simulink model "ControleFF_D_NL"  (R2020b)
settings: Solver=FixedStepAuto  StartTime=0  StopTime=10  FixedStep=1e-3  RelTol=1e-3
values from neighbouring files (symbols this model uses):
  alpha = alpha_vec(l)    [kermani_parameters.m]    (also in teste_controle_nao_linear.m = 1.25)
  Beff = 1    [kermani_parameters.m]    (also in teste_controle_nao_linear.m = 50)
  Fc = Fc_vec(k)    [kermani_parameters.m]    (also in teste_controle_nao_linear.m = 2173.5)
  Fs = Fs_vec(j)    [kermani_parameters.m]    (also in teste_controle_nao_linear.m = 2673.5)
  Jeff = 0.5    [kermani_parameters.m]    (also in teste_controle_nao_linear.m)
  K = (90/12)*(2*pi/60)    (= 0.785398163397)    [kermani_parameters.m]    (also in teste_controle_nao_linear.m)
  Kd = (2*xi*wn*Jeff - Beff)/K    (= 17.8253536263)    [kermani_parameters.m]    (also in teste_controle_nao_linear.m = -44.5633840657)
  Kp = (wn^2*Jeff)/K    (= 143.239448783)    [kermani_parameters.m]    (also in teste_controle_nao_linear.m)
  N = 3    [kermani_parameters.m]    (also in teste_controle_nao_linear.m)
  phi = 43.47    [teste_controle_nao_linear.m]
  r = 1./[231.22*4 139.138 139.138 231.22 231.22]    [kermani_parameters.m]    (also in teste_controle_nao_linear.m)
  sigma0 = sigma0_vec(m)    [kermani_parameters.m]    (also in teste_controle_nao_linear.m = 10000)
  sigma1 = sigma1_vec(n)    [kermani_parameters.m]    (also in teste_controle_nao_linear.m = 1000)
  sigma2 = sigma2_vec(o)    [kermani_parameters.m]    (also in teste_controle_nao_linear.m = 10)
libraries: simulink_extras x21
(part 11 of 14)

== matlab function ControleFF_D_NL/Dinâmica do robô2/Perturbação/V1 ==
  data: Th input; V output; dTh input
function V = calcul_V(Th, dTh)

th1 = Th(1);
th2 = Th(2);
th3 = Th(3);
th4 = Th(4);
th5 = Th(5);
dth1 = dTh(1);
dth2 = dTh(2);
dth3 = dTh(3);
dth4 = dTh(4);
dth5 = dTh(5);

V = [((217*cos(th2)*cos(th3)*cos(th4)*sin(th4))/80000 - (217*cos(th4)*sin(th2)*sin(th3)*sin(th4))/80000 + (87*cos(th2)*sin(th3)*sin(th4)*sin(th5))/5000 + (87*cos(th3)*sin(th2)*sin(th4)*sin(th5))/5000 + (9*cos(th2)*cos(th5)*sin(th3)*sin(th4)*sin(th5))/3200 + (9*cos(th3)*cos(th5)*sin(th2)*sin(th4)*sin(th5))/3200 - (9*cos(th2)*cos(th3)*cos(th4)*cos(th5)^2*sin(th4))/3200 + (9*cos(th4)*cos(th5)^2*sin(th2)*sin(th3)*sin(th4))/3200)*dth3^2 + ((217*cos(th2)*cos(th3)*cos(th4)*sin(th4))/80000 - (3*cos(th2)*sin(th4)*sin(th5))/160 - (217*cos(th4)*sin(th2)*sin(th3)*sin(th4))/80000 + (87*cos(th2)*sin(th3)*sin(th4)*sin(th5))/5000 + (87*cos(th3)*sin(th2)*sin(th4)*sin(th5))/5000 + (9*cos(th2)*cos(th5)*sin(th3)*sin(th4)*sin(th5))/3200 + (9*cos(th3)*cos(th5)*sin(th2)*sin(th4)*sin(th5))/3200 - (9*cos(th2)*cos(th3)*cos(th4)*cos(th5)^2*sin(th4))/3200 + (9*cos(th4)*cos(th5)^2*sin(th2)*sin(th3)*sin(th4))/3200)*dth2^2 + ((217*cos(th2)*cos(th4)^2*sin(th3))/40000 - (353*cos(th3)*sin(th2))/40000 - (353*cos(th2)*sin(th3))/40000 + (217*cos(th3)*cos(th4)^2*sin(th2))/40000 + (9*cos(th2)*cos(th5)^2*sin(th3))/1600 + (9*cos(th3)*cos(th5)^2*sin(th2))/1600 - (9*cos(th2)*cos(th4)^2*cos(th5)^2*sin(th3))/1600 - (9*cos(th3)*cos(th4)^2*cos(th5)^2*sin(th2))/1600)*dth2*dth4 + ((217*cos(th2)*cos(th4)^2*sin(th3))/40000 - (353*cos(th3)*sin(th2))/40000 - (353*cos(th2)*sin(th3))/40000 + (217*cos(th3)*cos(th4)^2*sin(th2))/40000 + (9*cos(th2)*cos(th5)^2*sin(th3))/1600 + (9*cos(th3)*cos(th5)^2*sin(th2))/1600 - (9*cos(th2)*cos(th4)^2*cos(th5)^2*sin(th3))/1600 - (9*cos(th3)*cos(th4)^2*cos(th5)^2*sin(th2))/1600)*dth3*dth4 + ((217*cos(th2)*cos(th3)*cos(th4)*sin(th4))/40000 - (217*cos(th4)*sin(th2)*sin(th3)*sin(th4))/40000 + (87*cos(th2)*sin(th3)*sin(th4)*sin(th5))/2500 + (87*cos(th3)*sin(th2)*sin(th4)*sin(th5))/2500 + (9*cos(th2)*cos(th5)*sin(th3)*sin(th4)*sin(th5))/1600 + (9*cos(th3)*cos(th5)*sin(th2)*sin(th4)*sin(th5))/1600 - (9*cos(th2)*cos(th3)*cos(th4)*cos(th5)^2*sin(th4))/1600 + (9*cos(th4)*cos(th5)^2*sin(th2)*sin(th3)*sin(th4))/1600)*dth2*dth3 + ((217*cos(th2)^2*cos(th4)*sin(th4))/40000 + (217*cos(th3)^2*cos(th4)*sin(th4))/40000 + (3*cos(th2)^2*cos(th3)*sin(th4)*sin(th5))/80 - (217*cos(th2)^2*cos(th3)^2*cos(th4)*sin(th4))/20000 - (9*cos(th2)^2*cos(th4)*cos(th5)^2*sin(th4))/1600 - (9*cos(th3)^2*cos(th4)*cos(th5)^2*sin(th4))/1600 + (87*cos(th2)*sin(th2)*sin(th4)*sin(th5))/2500 + (87*cos(th3)*sin(th3)*sin(th4)*sin(th5))/2500 + (9*cos(th2)^2*cos(th3)^2*cos(th4)*cos(th5)^2*sin(th4))/800 + (9*cos(th2)*cos(th5)*sin(th2)*sin(th4)*sin(th5))/1600 + (9*cos(th3)*cos(th5)*sin(th3)*sin(th4)*sin(th5))/1600 - (3*cos(th2)*sin(th2)*sin(th3)*sin(th4)*sin(th5))/80 - (87*cos(th2)*cos(th3)^2*sin(th2)*sin(th4)*sin(th5))/1250 - (87*cos(th2)^2*cos(th3)*sin(th3)*sin(th4)*sin(th5))/1250 + (217*cos(th2)*cos(th3)*cos(th4)*sin(th2)*sin(th3)*sin(th4))/20000 - (9*cos(th2)*cos(th3)^2*cos(th5)*sin(th2)*sin(th4)*sin(th5))/800 - (9*cos(th2)^2*cos(th3)*cos(th5)*sin(th3)*sin(th4)*sin(th5))/800 - (9*cos(th2)*cos(th3)*cos(th4)*cos(th5)^2*sin(th2)*sin(th3)*sin(th4))/800)*dth1*dth4 + ((87*cos(th4)*sin(th5))/2500 - (8453*sin(2*th3))/31250 - (8453*sin(2*th2))/31250 - (33*cos(th2)^2*cos(th3))/50 - (87*cos(th2)*cos(th5)*sin(th2))/1250 - (87*cos(th3)*cos(th5)*sin(th3))/1250 + (9*cos(th4)*cos(th5)*sin(th5))/1600 + (33*cos(th2)*sin(th2)*sin(th3))/50 - (3*cos(th2)^2*cos(th3)*cos(th5))/80 + (16906*cos(th2)*cos(th3)^2*sin(th2))/15625 + (217*cos(th2)*cos(th4)^2*sin(th2))/40000 + (16906*cos(th2)^2*cos(th3)*sin(th3))/15625 - (9*cos(th2)*cos(th5)^2*sin(th2))/1600 + (217*cos(th3)*cos(th4)^2*sin(th3))/40000 - (9*cos(th3)*cos(th5)^2*sin(th3))/1600 - (87*cos(th2)^2*cos(th4)*sin(th5))/1250 - (87*cos(th3)^2*cos(th4)*sin(th5))/1250 + (3*cos(th2)^2*cos(th4)*sin(th3)*sin(th5))/80 - (217*cos(th2)*cos(th3)^2*cos(th4)^2*sin(th2))/20000 + (9*cos(th2)*cos(th3)^2*cos(th5)^2*sin(th2))/800 - (217*cos(th2)^2*cos(th3)*cos(th4)^2*sin(th3))/20000 - (9*cos(th2)*cos(th4)^2*cos(th5)^2*sin(th2))/1600 + (9*cos(th2)^2*cos(th3)*cos(th5)^2*sin(th3))/800 + (87*cos(th2)^2*cos(th3)^2*cos(th4)*sin(th5))/625 - (9*cos(th3)*cos(th4)^2*cos(th5)^2*sin(th3))/1600 + (3*cos(th2)*cos(th5)*sin(th2)*sin(th3))/80 + (87*cos(th2)*cos(th3)^2*cos(th5)*sin(th2))/625 + (87*cos(th2)^2*cos(th3)*cos(th5)*sin(th3))/625 - (9*cos(th2)^2*cos(th4)*cos(th5)*sin(th5))/800 - (9*cos(th3)^2*cos(th4)*cos(th5)*sin(th5))/800 + (9*cos(th2)*cos(th3)^2*cos(th4)^2*cos(th5)^2*sin(th2))/800 + (9*cos(th2)^2*cos(th3)*cos(th4)^2*cos(th5)^2*sin(th3))/800 + (9*cos(th2)^2*cos(th3)^2*cos(th4)*cos(th5)*sin(th5))/400 + (3*cos(th2)*cos(th3)*cos(th4)*sin(th2)*sin(th5))/80 - (87*cos(th2)*cos(th3)*cos(th4)*sin(th2)*sin(th3)*sin(th5))/625 - (9*cos(th2)*cos(th3)*cos(th4)*cos(th5)*sin(th2)*sin(th3)*sin(th5))/400)*dth1*dth3 + ((33*cos(th3))/50 - (53231*sin(2*th2))/62500 - (8453*sin(2*th3))/31250 + (87*cos(th4)*sin(th5))/2500 - (33*cos(th2)^2*cos(th3))/25 + (3*cos(th3)*cos(th5))/80 - (87*cos(th2)*cos(th5)*sin(th2))/1250 - (87*cos(th3)*cos(th5)*sin(th3))/1250 + (9*cos(th4)*cos(th5)*sin(th5))/1600 + (33*cos(th2)*sin(th2)*sin(th3))/25 - (3*cos(th4)*sin(th3)*sin(th5))/80 - (3*cos(th2)^2*cos(th3)*cos(th5))/40 + (16906*cos(th2)*cos(th3)^2*sin(th2))/15625 + (217*cos(th2)*cos(th4)^2*sin(th2))/40000 + (16906*cos(th2)^2*cos(th3)*sin(th3))/15625 - (9*cos(th2)*cos(th5)^2*sin(th2))/1600 + (217*cos(th3)*cos(th4)^2*sin(th3))/40000 - (9*cos(th3)*cos(th5)^2*sin(th3))/1600 - (87*cos(th2)^2*cos(th4)*sin(th5))/1250 - (87*cos(th3)^2*cos(th4)*sin(th5))/1250 + (3*cos(th2)^2*cos(th4)*sin(th3)*sin(th5))/40 - (217*cos(th2)*cos(th3)^2*cos(th4)^2*sin(th2))/20000 + (9*cos(th2)*cos(th3)^2*cos(th5)^2*sin(th2))/800 - (217*cos(th2)^2*cos(th3)*cos(th4)^2*sin(th3))/20000 - (9*cos(th2)*cos(th4)^2*cos(th5)^2*sin(th2))/1600 + (9*cos(th2)^2*cos(th3)*cos(th5)^2*sin(th3))/800 + (87*cos(th2)^2*cos(th3)^2*cos(th4)*sin(th5))/625 - (9*cos(th3)*cos(th4)^2*cos(th5)^2*sin(th3))/1600 + (3*cos(th2)*cos(th5)*sin(th2)*sin(th3))/40 + (87*cos(th2)*cos(th3)^2*cos(th5)*sin(th2))/625 + (87*cos(th2)^2*cos(th3)*cos(th5)*sin(th3))/625 - (9*cos(th2)^2*cos(th4)*cos(th5)*sin(th5))/800 - (9*cos(th3)^2*cos(th4)*cos(th5)*sin(th5))/800 + (9*cos(th2)*cos(th3)^2*cos(th4)^2*cos(th5)^2*sin(th2))/800 + (9*cos(th2)^2*cos(th3)*cos(th4)^2*cos(th5)^2*sin(th3))/800 + (9*cos(th2)^2*cos(th3)^2*cos(th4)*cos(th5)*sin(th5))/400 + (3*cos(th2)*cos(th3)*cos(th4)*sin(th2)*sin(th5))/40 - (87*cos(th2)*cos(th3)*cos(th4)*sin(th2)*sin(th3)*sin(th5))/625 - (9*cos(th2)*cos(th3)*cos(th4)*cos(th5)*sin(th2)*sin(th3)*sin(th5))/400)*dth1*dth2 + ((3*cos(th2)*sin(th4)*sin(th5))/160 - (87*cos(th2)*sin(th3)*sin(th4)*sin(th5))/5000 - (87*cos(th3)*sin(th2)*sin(th4)*sin(th5))/5000)*dth5^2 + ((3*cos(th2)*sin(th4)*sin(th5))/160 - (87*cos(th2)*sin(th3)*sin(th4)*sin(th5))/5000 - (87*cos(th3)*sin(th2)*sin(th4)*sin(th5))/5000 - (9*cos(th2)*cos(th5)*sin(th3)*sin(th4)*sin(th5))/3200 - (9*cos(th3)*cos(th5)*sin(th2)*sin(th4)*sin(th5))/3200)*dth4^2 + ((cos(th2)*cos(th4)*sin(th3))/625 - (3*cos(th2)*cos(th4)*cos(th5))/80 + (cos(th3)*cos(th4)*sin(th2))/625 + (87*cos(th2)*cos(th4)*cos(th5)*sin(th3))/2500 + (87*cos(th3)*cos(th4)*cos(th5)*sin(th2))/2500 + (9*cos(th2)*cos(th3)*cos(th5)*sin(th5))/1600 - (9*cos(th5)*sin(th2)*sin(th3)*sin(th5))/1600 + (9*cos(th2)*cos(th4)*cos(th5)^2*sin(th3))/1600 + (9*cos(th3)*cos(th4)*cos(th5)^2*sin(th2))/1600)*dth4*dth5 + ((289*cos(th2)*cos(th3)*sin(th4))/40000 - (289*sin(th2)*sin(th3)*sin(th4))/40000 + (9*cos(th5)^2*sin(th2)*sin(th3)*sin(th4))/1600 - (9*cos(th2)*cos(th3)*cos(th5)^2*sin(th4))/1600 + (9*cos(th2)*cos(th4)*cos(th5)*sin(th3)*sin(th4)*sin(th5))/1600 + (9*cos(th3)*cos(th4)*cos(th5)*sin(th2)*sin(th4)*sin(th5))/1600)*dth2*dth5 + ((289*cos(th2)*cos(th3)*sin(th4))/40000 - (289*sin(th2)*sin(th3)*sin(th4))/40000 + (9*cos(th5)^2*sin(th2)*sin(th3)*sin(th4))/1600 - (9*cos(th2)*cos(th3)*cos(th5)^2*sin(th4))/1600 + (9*cos(th2)*cos(th4)*cos(th5)*sin(th3)*sin(th4)*sin(th5))/1600 + (9*cos(th3)*cos(th4)*cos(th5)*sin(th2)*sin(th4)*sin(th5))/1600)*dth3*dth5 + ((9*sin(2*th5))/3200 - (87*cos(th2)^2*sin(th5))/2500 - (87*cos(th3)^2*sin(th5))/2500 + (87*cos(th2)^2*cos(th3)^2*sin(th5))/1250 + (9*cos(th2)*cos(th4)*sin(th2))/1600 + (9*cos(th3)*cos(th4)*sin(th3))/1600 - (9*cos(th2)^2*cos(th5)*sin(th5))/1600 - (9*cos(th3)^2*cos(th5)*sin(th5))/1600 + (3*cos(th2)^2*sin(th3)*sin(th5))/80 + (9*cos(th2)^2*cos(th3)^2*cos(th5)*sin(th5))/800 - (9*cos(th2)^2*cos(th4)^2*cos(th5)*sin(th5))/1600 - (9*cos(th3)^2*cos(th4)^2*cos(th5)*sin(th5))/1600 - (87*cos(th2)*cos(th4)*cos(th5)*sin(th2))/2500 - (87*cos(th3)*cos(th4)*cos(th5)*sin(th3))/2500 + (3*cos(th2)*cos(th3)*sin(th2)*sin(th5))/80 - (3*cos(th2)^2*cos(th3)*cos(th4)*cos(th5))/80 - (9*cos(th2)*cos(th3)^2*cos(th4)*sin(th2))/800 - (9*cos(th2)^2*cos(th3)*cos(th4)*sin(th3))/800 - (9*cos(th2)*cos(th4)*cos(th5)^2*sin(th2))/800 - (9*cos(th3)*cos(th4)*cos(th5)^2*sin(th3))/800 + (9*cos(th2)^2*cos(th3)^2*cos(th4)^2*cos(th5)*sin(th5))/800 - (87*cos(th2)*cos(th3)*sin(th2)*sin(th3)*sin(th5))/1250 + (87*cos(th2)*cos(th3)^2*cos(th4)*cos(th5)*sin(th2))/1250 + (87*cos(th2)^2*cos(th3)*cos(th4)*cos(th5)*sin(th3))/1250 + (9*cos(th2)*cos(th3)^2*cos(th4)*cos(th5)^2*sin(th2))/400 + (9*cos(th2)^2*cos(th3)*cos(th4)*cos(th5)^2*sin(th3))/400 + (3*cos(th2)*cos(th4)*cos(th5)*sin(th2)*sin(th3))/80 - (9*cos(th2)*cos(th3)*cos(th5)*sin(th2)*sin(th3)*sin(th5))/800 - (9*cos(th2)*cos(th3)*cos(th4)^2*cos(th5)*sin(th2)*sin(th3)*sin(th5))/800)*dth1*dth5;
                                                                                                                                                                                                                                                                                                                                                                                                                                                                                                                                                                                                                                                                                                                                                                                                                                                                                                                                                                                                                                                                                                                                                                                                                                                                                                                                                                                                                                                                                                                                                                                                                                                                                                                                                                                                                                                                                                                                                                                                                                                                                                                                                                                                                                                                                                                                                                                                                                                                                                                                                                                                                                                                                                                                                                                                                                                                                                                                                                                                                                                                                                                                                                                                                                                                                                                                                                                                                                                                                                                                                                                                                                                                                                                                                                                                                                                                                                                                                                                                                                                                                                                                                                                                                                                                                                                                                                                                                                                                                                                                                                                                                                                                                                                                                                                                                                                                                                                                                                                                                                                                                                                                                                                                                                                                                                                                                                                                                                                                                                                                                                                                                                                                                                                                                                                                                                                                                                                                                                                                                                                                                                                                                                                                                                                                                                                                                                                                                                                                                                                                                                                                                                                                                                                                                                                                                                                                                                                                                                                                                                                                                                                                                                                                                                  ((53231*sin(2*th2))/125000 - (33*cos(th3))/100 + (8453*sin(2*th3))/62500 - (87*cos(th4)*sin(th5))/5000 + (33*cos(th2)^2*cos(th3))/50 - (3*cos(th3)*cos(th5))/160 + (87*cos(th2)*cos(th5)*sin(th2))/2500 + (87*cos(th3)*cos(th5)*sin(th3))/2500 - (9*cos(th4)*cos(th5)*sin(th5))/3200 - (33*cos(th2)*sin(th2)*sin(th3))/50 + (3*cos(th4)*sin(th3)*sin(th5))/160 + (3*cos(th2)^2*cos(th3)*cos(th5))/80 - (8453*cos(th2)*cos(th3)^2*sin(th2))/15625 - (217*cos(th2)*cos(th4)^2*sin(th2))/80000 - (8453*cos(th2)^2*cos(th3)*sin(th3))/15625 + (9*cos(th2)*cos(th5)^2*sin(th2))/3200 - (217*cos(th3)*cos(th4)^2*sin(th3))/80000 + (9*cos(th3)*cos(th5)^2*sin(th3))/3200 + (87*cos(th2)^2*cos(th4)*sin(th5))/2500 + (87*cos(th3)^2*cos(th4)*sin(th5))/2500 - (3*cos(th2)^2*cos(th4)*sin(th3)*sin(th5))/80 + (217*cos(th2)*cos(th3)^2*cos(th4)^2*sin(th2))/40000 - (9*cos(th2)*cos(th3)^2*cos(th5)^2*sin(th2))/1600 + (217*cos(th2)^2*cos(th3)*cos(th4)^2*sin(th3))/40000 + (9*cos(th2)*cos(th4)^2*cos(th5)^2*sin(th2))/3200 - (9*cos(th2)^2*cos(th3)*cos(th5)^2*sin(th3))/1600 - (87*cos(th2)^2*cos(th3)^2*cos(th4)*sin(th5))/1250 + (9*cos(th3)*cos(th4)^2*cos(th5)^2*sin(th3))/3200 - (3*cos(th2)*cos(th5)*sin(th2)*sin(th3))/80 - (87*cos(th2)*cos(th3)^2*cos(th5)*sin(th2))/1250 - (87*cos(th2)^2*cos(th3)*cos(th5)*sin(th3))/1250 + (9*cos(th2)^2*cos(th4)*cos(th5)*sin(th5))/1600 + (9*cos(th3)^2*cos(th4)*cos(th5)*sin(th5))/1600 - (9*cos(th2)*cos(th3)^2*cos(th4)^2*cos(th5)^2*sin(th2))/1600 - (9*cos(th2)^2*cos(th3)*cos(th4)^2*cos(th5)^2*sin(th3))/1600 - (9*cos(th2)^2*cos(th3)^2*cos(th4)*cos(th5)*sin(th5))/800 - (3*cos(th2)*cos(th3)*cos(th4)*sin(th2)*sin(th5))/80 + (87*cos(th2)*cos(th3)*cos(th4)*sin(th2)*sin(th3)*sin(th5))/1250 + (9*cos(th2)*cos(th3)*cos(th4)*cos(th5)*sin(th2)*sin(th3)*sin(th5))/800)*dth1^2 + ((17*cos(th2)*sin(th3))/5000 + (17*cos(th3)*sin(th2))/5000 - (3*cos(th4)*sin(th2)*sin(th5))/80 + (217*cos(th2)*cos(th4)^2*sin(th3))/40000 + (217*cos(th3)*cos(th4)^2*sin(th2))/40000 - (9*cos(th2)*cos(th4)^2*cos(th5)^2*sin(th3))/1600 - (9*cos(th3)*cos(th4)^2*cos(th5)^2*sin(th2))/1600 - (87*cos(th2)*cos(th3)*cos(th4)*sin(th5))/2500 + (87*cos(th4)*sin(th2)*sin(th3)*sin(th5))/2500 + (9*cos(th4)*cos(th5)*sin(th2)*sin(th3)*sin(th5))/1600 - (9*cos(th2)*cos(th3)*cos(th4)*cos(th5)*sin(th5))/1600)*dth1*dth4 + ((3*cos(th4)*sin(th3)*sin(th5))/160 - (3*cos(th3)*cos(th5))/160 - (87*cos(th4)*sin(th5))/5000)*dth5^2 + ((9*cos(th4)*sin(th4)*cos(th5)^2)/1600 - (217*sin(2*th4))/80000 + (3*cos(th3)*sin(th4)*sin(th5))/80)*dth2*dth4 + ((9*cos(th4)*sin(th4)*cos(th5)^2)/1600 - (217*sin(2*th4))/80000 + (3*cos(th3)*sin(th4)*sin(th5))/80)*dth3*dth4 + ((3*cos(th4)*sin(th3)*sin(th5))/160 - (9*cos(th4)*cos(th5)*sin(th5))/3200 - (87*cos(th4)*sin(th5))/5000)*dth4^2 + ((sin(th2)*sin(th3)*sin(th4))/625 - (3*cos(th5)*sin(th2)*sin(th4))/80 - (cos(th2)*cos(th3)*sin(th4))/625 + (9*cos(th5)^2*sin(th2)*sin(th3)*sin(th4))/1600 - (87*cos(th2)*cos(th3)*cos(th5)*sin(th4))/2500 + (87*cos(th5)*sin(th2)*sin(th3)*sin(th4))/2500 - (9*cos(th2)*cos(th3)*cos(th5)^2*sin(th4))/1600 + (9*cos(th2)*cos(th4)*cos(th5)*sin(th3)*sin(th4)*sin(th5))/1600 + (9*cos(th3)*cos(th4)*cos(th5)*sin(th2)*sin(th4)*sin(th5))/1600)*dth1*dth5 + ((3*cos(th4)*sin(th3)*sin(th5))/160 - (3*cos(th3)*cos(th5))/160 - (33*cos(th3))/100)*dth3^2 + ((9*cos(th5)*sin(th5)*cos(th4)^2)/1600 - (3*cos(th3)*cos(th5)*cos(th4))/80 - (87*sin(th5))/2500 - (9*sin(2*th5))/3200 + (3*sin(th3)*sin(th5))/80)*dth2*dth5 + ((9*cos(th5)*sin(th5)*cos(th4)^2)/1600 - (3*cos(th3)*cos(th5)*cos(th4))/80 - (87*sin(th5))/2500 - (9*sin(2*th5))/3200 + (3*sin(th3)*sin(th5))/80)*dth3*dth5 + ((3*cos(th4)*sin(th3)*sin(th5))/80 - (3*cos(th3)*cos(th5))/80 - (33*cos(th3))/50)*dth2*dth3 + ((3*cos(th5)*sin(th3)*sin(th4))/80 - (87*cos(th5)*sin(th4))/2500 - (9*cos(th5)^2*sin(th4))/1600 - sin(th4)/625)*dth4*dth5;
                                                                                                                                                                                                                                                                                                                                                                                                                                                                                                                                                                                                                                                                                                                                                                                                                                                                                                                                                                                                                                                                                                                                                                                                                                                                                                                                                                                                                                                                                                                                                                                                                                                                                                                                                                                                                                                                                                                                                                                                                                                                                                                                                                                                                                                                                                                                                                                                                                                                                                                                                                                                                                                                                                                                                                                                                                                                                                                                                                                                                                                                                                                                                                                                                                                                                                                                                                                                                                                                                                                                                                                                                                                                                                                                                                                                                                                                                                                                                                                                                                                                                                                                                                                                                                                                                                                                                                                                                                                                                                                                                                                                                                                                                                                                                                                                                                                                                                                                                                                                                                                                                                                                                                                                                                                                                                                                                                                                                                                                                                                                                                                                                                                                                                                                                                                                                                                                                                                                                                                                                                                                                                                                                                                                                                                                                                                                                                                                                                                                                                                                                                                                                                                                                                                                                                                                                                                                                                                                                                                                                                                                                                                                                                                                                                                                                                                                                                                                                                                                                                                                                                                                                                                                                                                                                                                                                                                                                                                                                                                 ((8453*sin(2*th2))/62500 + (8453*sin(2*th3))/62500 - (87*cos(th4)*sin(th5))/5000 + (33*cos(th2)^2*cos(th3))/100 + (87*cos(th2)*cos(th5)*sin(th2))/2500 + (87*cos(th3)*cos(th5)*sin(th3))/2500 - (9*cos(th4)*cos(th5)*sin(th5))/3200 - (33*cos(th2)*sin(th2)*sin(th3))/100 + (3*cos(th2)^2*cos(th3)*cos(th5))/160 - (8453*cos(th2)*cos(th3)^2*sin(th2))/15625 - (217*cos(th2)*cos(th4)^2*sin(th2))/80000 - (8453*cos(th2)^2*cos(th3)*sin(th3))/15625 + (9*cos(th2)*cos(th5)^2*sin(th2))/3200 - (217*cos(th3)*cos(th4)^2*sin(th3))/80000 + (9*cos(th3)*cos(th5)^2*sin(th3))/3200 + (87*cos(th2)^2*cos(th4)*sin(th5))/2500 + (87*cos(th3)^2*cos(th4)*sin(th5))/2500 - (3*cos(th2)^2*cos(th4)*sin(th3)*sin(th5))/160 + (217*cos(th2)*cos(th3)^2*cos(th4)^2*sin(th2))/40000 - (9*cos(th2)*cos(th3)^2*cos(th5)^2*sin(th2))/1600 + (217*cos(th2)^2*cos(th3)*cos(th4)^2*sin(th3))/40000 + (9*cos(th2)*cos(th4)^2*cos(th5)^2*sin(th2))/3200 - (9*cos(th2)^2*cos(th3)*cos(th5)^2*sin(th3))/1600 - (87*cos(th2)^2*cos(th3)^2*cos(th4)*sin(th5))/1250 + (9*cos(th3)*cos(th4)^2*cos(th5)^2*sin(th3))/3200 - (3*cos(th2)*cos(th5)*sin(th2)*sin(th3))/160 - (87*cos(th2)*cos(th3)^2*cos(th5)*sin(th2))/1250 - (87*cos(th2)^2*cos(th3)*cos(th5)*sin(th3))/1250 + (9*cos(th2)^2*cos(th4)*cos(th5)*sin(th5))/1600 + (9*cos(th3)^2*cos(th4)*cos(th5)*sin(th5))/1600 - (9*cos(th2)*cos(th3)^2*cos(th4)^2*cos(th5)^2*sin(th2))/1600 - (9*cos(th2)^2*cos(th3)*cos(th4)^2*cos(th5)^2*sin(th3))/1600 - (9*cos(th2)^2*cos(th3)^2*cos(th4)*cos(th5)*sin(th5))/800 - (3*cos(th2)*cos(th3)*cos(th4)*sin(th2)*sin(th5))/160 + (87*cos(th2)*cos(th3)*cos(th4)*sin(th2)*sin(th3)*sin(th5))/1250 + (9*cos(th2)*cos(th3)*cos(th4)*cos(th5)*sin(th2)*sin(th3)*sin(th5))/800)*dth1^2 + ((33*cos(th3))/100 + (3*cos(th3)*cos(th5))/160 - (3*cos(th4)*sin(th3)*sin(th5))/160)*dth2^2 + ((9*cos(th4)*cos(th5)^2*sin(th4))/1600 - (217*sin(2*th4))/80000)*dth2*dth4 + ((9*cos(th4)*cos(th5)^2*sin(th4))/1600 - (217*sin(2*th4))/80000)*dth3*dth4 + (- (87*cos(th4)*sin(th5))/5000 - (9*cos(th4)*cos(th5)*sin(th5))/3200)*dth4^2 + ((sin(th2)*sin(th3)*sin(th4))/625 - (cos(th2)*cos(th3)*sin(th4))/625 + (9*cos(th5)^2*sin(th2)*sin(th3)*sin(th4))/1600 - (87*cos(th2)*cos(th3)*cos(th5)*sin(th4))/2500 + (87*cos(th5)*sin(th2)*sin(th3)*sin(th4))/2500 - (9*cos(th2)*cos(th3)*cos(th5)^2*sin(th4))/1600 + (9*cos(th2)*cos(th4)*cos(th5)*sin(th3)*sin(th4)*sin(th5))/1600 + (9*cos(th3)*cos(th4)*cos(th5)*sin(th2)*sin(th4)*sin(th5))/1600)*dth1*dth5 + (-(87*cos(th4)*sin(th5))/5000)*dth5^2 + ((17*cos(th2)*sin(th3))/5000 + (17*cos(th3)*sin(th2))/5000 + (217*cos(th2)*cos(th4)^2*sin(th3))/40000 + (217*cos(th3)*cos(th4)^2*sin(th2))/40000 - (9*cos(th2)*cos(th4)^2*cos(th5)^2*sin(th3))/1600 - (9*cos(th3)*cos(th4)^2*cos(th5)^2*sin(th2))/1600 - (87*cos(th2)*cos(th3)*cos(th4)*sin(th5))/2500 + (87*cos(th4)*sin(th2)*sin(th3)*sin(th5))/2500 + (9*cos(th4)*cos(th5)*sin(th2)*sin(th3)*sin(th5))/1600 - (9*cos(th2)*cos(th3)*cos(th4)*cos(th5)*sin(th5))/1600)*dth1*dth4 + (- (9*sin(th4)*cos(th5)^2)/1600 - (87*sin(th4)*cos(th5))/2500 - sin(th4)/625)*dth4*dth5 + ((9*cos(th5)*sin(th5)*cos(th4)^2)/1600 - (87*sin(th5))/2500 - (9*sin(2*th5))/3200)*dth2*dth5 + ((9*cos(th5)*sin(th5)*cos(th4)^2)/1600 - (87*sin(th5))/2500 - (9*sin(2*th5))/3200)*dth3*dth5;
                                                                                                                                                                                                                                                                                                                                                                                                                                                                                                                                                                                                                                                                                                                                                                                                                                                                                                                                                                                                                                                                                                                                                                                                                                                                                                                                                                                                                                                                                                                                                                                                                                                                                                                                                                                                                                                                                                                                                                                                                                                                                                                                                                                                                                                                                                                                                                                                                                                                                                                                                                                                                                                                                                                                                                                                                                                                                                                                                                                                                                                                                                                                                                                                                                                                                                                                                                                                                                                                                                                                                                                                                                                                                                                                                                                                                                                                                                                                                                                                                                                                                                                                                                                                                                                                                                                                                                                                                                                                                                                                                                                                                                                                                                                                                                                                                                                                                                                                                                                                                                                                                                                                                                                                                                                                                                                                                                                                                                                                                                                                                                                                                                                                                                                                                                                                                                                                                                                                                                                                                                                                                                                                                                                                                                                                                                                                                                                                                                                                                                                                                                                                                                                                                                                                                                                                                                                                                                                                                                                                                                                                                                                                                                                                                                                                                                                                                                                                                                                                                                                                                                                                                                                                                                                                                                                                                                                                                                                                                                                                                                                                                                                                                                                                                                                                                                                                                                                                                                                                                                                                                                                                     ((217*sin(2*th4))/160000 - (9*cos(th4)*cos(th5)^2*sin(th4))/3200)*dth3^2 + ((217*cos(th2)^2*cos(th3)^2*cos(th4)*sin(th4))/40000 - (217*cos(th3)^2*cos(th4)*sin(th4))/80000 - (3*cos(th2)^2*cos(th3)*sin(th4)*sin(th5))/160 - (217*cos(th2)^2*cos(th4)*sin(th4))/80000 + (9*cos(th2)^2*cos(th4)*cos(th5)^2*sin(th4))/3200 + (9*cos(th3)^2*cos(th4)*cos(th5)^2*sin(th4))/3200 - (87*cos(th2)*sin(th2)*sin(th4)*sin(th5))/5000 - (87*cos(th3)*sin(th3)*sin(th4)*sin(th5))/5000 - (9*cos(th2)^2*cos(th3)^2*cos(th4)*cos(th5)^2*sin(th4))/1600 - (9*cos(th2)*cos(th5)*sin(th2)*sin(th4)*sin(th5))/3200 - (9*cos(th3)*cos(th5)*sin(th3)*sin(th4)*sin(th5))/3200 + (3*cos(th2)*sin(th2)*sin(th3)*sin(th4)*sin(th5))/160 + (87*cos(th2)*cos(th3)^2*sin(th2)*sin(th4)*sin(th5))/2500 + (87*cos(th2)^2*cos(th3)*sin(th3)*sin(th4)*sin(th5))/2500 - (217*cos(th2)*cos(th3)*cos(th4)*sin(th2)*sin(th3)*sin(th4))/40000 + (9*cos(th2)*cos(th3)^2*cos(th5)*sin(th2)*sin(th4)*sin(th5))/1600 + (9*cos(th2)^2*cos(th3)*cos(th5)*sin(th3)*sin(th4)*sin(th5))/1600 + (9*cos(th2)*cos(th3)*cos(th4)*cos(th5)^2*sin(th2)*sin(th3)*sin(th4))/1600)*dth1^2 + ((217*sin(2*th4))/160000 - (9*cos(th4)*sin(th4)*cos(th5)^2)/3200 - (3*cos(th3)*sin(th4)*sin(th5))/160)*dth2^2 + ((9*sin(2*th5))/3200)*dth4*dth5 + ((217*sin(2*th4))/80000 - (9*cos(th4)*cos(th5)^2*sin(th4))/1600)*dth2*dth3 + ((9*cos(th2)*cos(th3)*cos(th5)*sin(th5))/1600 - (289*cos(th3)*cos(th4)*sin(th2))/40000 - (289*cos(th2)*cos(th4)*sin(th3))/40000 - (9*cos(th5)*sin(th2)*sin(th3)*sin(th5))/1600 + (9*cos(th2)*cos(th4)*cos(th5)^2*sin(th3))/1600 + (9*cos(th3)*cos(th4)*cos(th5)^2*sin(th2))/1600)*dth1*dth5 + ((289*sin(th4))/40000 - (9*cos(th5)^2*sin(th4))/1600)*dth2*dth5 + ((289*sin(th4))/40000 - (9*cos(th5)^2*sin(th4))/1600)*dth3*dth5 + ((3*cos(th4)*sin(th2)*sin(th5))/80 - (17*cos(th3)*sin(th2))/5000 - (17*cos(th2)*sin(th3))/5000 - (217*cos(th2)*cos(th4)^2*sin(th3))/40000 - (217*cos(th3)*cos(th4)^2*sin(th2))/40000 + (9*cos(th2)*cos(th4)^2*cos(th5)^2*sin(th3))/1600 + (9*cos(th3)*cos(th4)^2*cos(th5)^2*sin(th2))/1600 + (87*cos(th2)*cos(th3)*cos(th4)*sin(th5))/2500 - (87*cos(th4)*sin(th2)*sin(th3)*sin(th5))/2500 - (9*cos(th4)*cos(th5)*sin(th2)*sin(th3)*sin(th5))/1600 + (9*cos(th2)*cos(th3)*cos(th4)*cos(th5)*sin(th5))/1600)*dth1*dth2 + ((9*cos(th2)*cos(th4)^2*cos(th5)^2*sin(th3))/1600 - (17*cos(th3)*sin(th2))/5000 - (217*cos(th2)*cos(th4)^2*sin(th3))/40000 - (217*cos(th3)*cos(th4)^2*sin(th2))/40000 - (17*cos(th2)*sin(th3))/5000 + (9*cos(th3)*cos(th4)^2*cos(th5)^2*sin(th2))/1600 + (87*cos(th2)*cos(th3)*cos(th4)*sin(th5))/2500 - (87*cos(th4)*sin(th2)*sin(th3)*sin(th5))/2500 - (9*cos(th4)*cos(th5)*sin(th2)*sin(th3)*sin(th5))/1600 + (9*cos(th2)*cos(th3)*cos(th4)*cos(th5)*sin(th5))/1600)*dth1*dth3;
                                                                                                                                                                                                                                                                                                                                                                                                                                                                                                                                                                                                                                                                                                                                                                                                                                                                                                                                                                                                                                                                                                                                                                                                                                                                                                                                                                                                                                                                                                                                                                                                                                                                                                                                                                                                                                                                                                                                                                                                                                                                                                                                                                                                                                                                                                                                                                                                                                                                                                                                                                                                                                                                                                                                                                                                                                                                                                                                                                                                                                                                                                                                                                                                                                                                                                                                                                                                                                                                                                                                                                                                                                                                                                                                                                                                                                                                                                                                                                                                                                                                                                                                                                                                                                                                                                                                                                                                                                                                                                                                                                                                                                                                                                                                                                                                                                                                                                                                                                                                                                                                                                                                                                                                                                                                                                                                                                                                                                                                                                                                                                                                                                                                                                                                                                                                                                                                                                                                                                                                                                                                                                                                                                                                                                                                                                                                                                                                                                                                                                                                                                                                                                                                                                                                                                                                                                                                                                                                                                                                                                                                                                                                                                                                                                                                                                                                                                                                                                                                                                                                                                                                                                                                                                                                                                                                                                                                                                                                                                                                                                                                                                                                      ((87*sin(th5))/5000 - (9*cos(th5)*sin(th5)*cos(th4)^2)/3200 + (9*sin(2*th5))/6400)*dth3^2 + ((3*cos(th3)*cos(th5)*cos(th4))/160 - (9*cos(th5)*sin(th5)*cos(th4)^2)/3200 + (87*sin(th5))/5000 + (9*sin(2*th5))/6400 - (3*sin(th3)*sin(th5))/160)*dth2^2 + ((87*cos(th2)^2*sin(th5))/5000 - (9*sin(2*th5))/6400 + (87*cos(th3)^2*sin(th5))/5000 - (87*cos(th2)^2*cos(th3)^2*sin(th5))/2500 - (9*cos(th2)*cos(th4)*sin(th2))/3200 - (9*cos(th3)*cos(th4)*sin(th3))/3200 + (9*cos(th2)^2*cos(th5)*sin(th5))/3200 + (9*cos(th3)^2*cos(th5)*sin(th5))/3200 - (3*cos(th2)^2*sin(th3)*sin(th5))/160 - (9*cos(th2)^2*cos(th3)^2*cos(th5)*sin(th5))/1600 + (9*cos(th2)^2*cos(th4)^2*cos(th5)*sin(th5))/3200 + (9*cos(th3)^2*cos(th4)^2*cos(th5)*sin(th5))/3200 + (87*cos(th2)*cos(th4)*cos(th5)*sin(th2))/5000 + (87*cos(th3)*cos(th4)*cos(th5)*sin(th3))/5000 - (3*cos(th2)*cos(th3)*sin(th2)*sin(th5))/160 + (3*cos(th2)^2*cos(th3)*cos(th4)*cos(th5))/160 + (9*cos(th2)*cos(th3)^2*cos(th4)*sin(th2))/1600 + (9*cos(th2)^2*cos(th3)*cos(th4)*sin(th3))/1600 + (9*cos(th2)*cos(th4)*cos(th5)^2*sin(th2))/1600 + (9*cos(th3)*cos(th4)*cos(th5)^2*sin(th3))/1600 - (9*cos(th2)^2*cos(th3)^2*cos(th4)^2*cos(th5)*sin(th5))/1600 + (87*cos(th2)*cos(th3)*sin(th2)*sin(th3)*sin(th5))/2500 - (87*cos(th2)*cos(th3)^2*cos(th4)*cos(th5)*sin(th2))/2500 - (87*cos(th2)^2*cos(th3)*cos(th4)*cos(th5)*sin(th3))/2500 - (9*cos(th2)*cos(th3)^2*cos(th4)*cos(th5)^2*sin(th2))/800 - (9*cos(th2)^2*cos(th3)*cos(th4)*cos(th5)^2*sin(th3))/800 - (3*cos(th2)*cos(th4)*cos(th5)*sin(th2)*sin(th3))/160 + (9*cos(th2)*cos(th3)*cos(th5)*sin(th2)*sin(th3)*sin(th5))/1600 + (9*cos(th2)*cos(th3)*cos(th4)^2*cos(th5)*sin(th2)*sin(th3)*sin(th5))/1600)*dth1^2 + ((289*cos(th2)*cos(th4)*sin(th3))/40000 + (289*cos(th3)*cos(th4)*sin(th2))/40000 - (9*cos(th2)*cos(th3)*cos(th5)*sin(th5))/1600 + (9*cos(th5)*sin(th2)*sin(th3)*sin(th5))/1600 - (9*cos(th2)*cos(th4)*cos(th5)^2*sin(th3))/1600 - (9*cos(th3)*cos(th4)*cos(th5)^2*sin(th2))/1600)*dth1*dth4 + ((9*cos(th5)^2*sin(th4))/1600 - (289*sin(th4))/40000)*dth2*dth4 + ((9*cos(th5)^2*sin(th4))/1600 - (289*sin(th4))/40000)*dth3*dth4 + (-(9*sin(2*th5))/6400)*dth4^2 + ((87*sin(th5))/2500 - (9*cos(th5)*sin(th5)*cos(th4)^2)/1600 + (9*sin(2*th5))/3200)*dth2*dth3 + ((cos(th2)*cos(th3)*sin(th4))/625 - (sin(th2)*sin(th3)*sin(th4))/625 - (9*cos(th5)^2*sin(th2)*sin(th3)*sin(th4))/1600 + (87*cos(th2)*cos(th3)*cos(th5)*sin(th4))/2500 - (87*cos(th5)*sin(th2)*sin(th3)*sin(th4))/2500 + (9*cos(th2)*cos(th3)*cos(th5)^2*sin(th4))/1600 - (9*cos(th2)*cos(th4)*cos(th5)*sin(th3)*sin(th4)*sin(th5))/1600 - (9*cos(th3)*cos(th4)*cos(th5)*sin(th2)*sin(th4)*sin(th5))/1600)*dth1*dth3 + ((cos(th2)*cos(th3)*sin(th4))/625 + (3*cos(th5)*sin(th2)*sin(th4))/80 - (sin(th2)*sin(th3)*sin(th4))/625 - (9*cos(th5)^2*sin(th2)*sin(th3)*sin(th4))/1600 + (87*cos(th2)*cos(th3)*cos(th5)*sin(th4))/2500 - (87*cos(th5)*sin(th2)*sin(th3)*sin(th4))/2500 + (9*cos(th2)*cos(th3)*cos(th5)^2*sin(th4))/1600 - (9*cos(th2)*cos(th4)*cos(th5)*sin(th3)*sin(th4)*sin(th5))/1600 - (9*cos(th3)*cos(th4)*cos(th5)*sin(th2)*sin(th4)*sin(th5))/1600)*dth1*dth2];
